simulink library "ammclib_bam"  (Simulink 9.3)
settings: Solver=VariableStepAuto  StartTime=0.0  StopTime=10.0  RelTol=1e-3
undefined symbols (not defined in the file or in its folder): f16A1, f16A2, f16ADCMaxError, f16B0, f16B1, f16B2, f16C1, f16CC1, f16CC1sc, f16CC1sc_D, f16CC1sc_Q, f16CC2, f16CC2sc, f16CC2sc_D, f16CC2sc_Q, f16DerivGain, f16EGain, f16FiltCoef, f16HystOff, f16HystOn, f16IGain, f16IntegGain, f16IntegGainFW, f16IntegGainQ, f16Kd, f16Kq, f16Limit, f16LowerLimit, f16LowerLimit_D, f16LowerLimit_Q, f16LowerLimitFW, f16LowerLimitQ, f16ModIndex, f16OutValOff, f16OutValOn, f16PropGain, f16PropGainFW, f16PropGainQ, f16RampDown, f16RampUp, f16UGain, f16UpperLimit, f16UpperLimit_D, f16UpperLimit_Q, f16UpperLimitFW, f16UpperLimitQ, f16WIGain, f32A1, f32A2, f32ADCMaxError, f32B0, f32B1, f32B2, f32C1, f32CC1, f32CC1sc, f32CC1sc_D, f32CC1sc_Q, f32CC2, f32CC2sc ... (+114)
(part 20 of 21)

== system ammclib_bam/MLIB/F16/MLIB_ShLSat_F16 ==
  f16In1 : Inport  OutDataTypeStr=int16
  u16In2 : Inport  Port=2  OutDataTypeStr=uint16
  MLIB_ShLSat_SF : S-Function  FunctionName=MLIB_ShLSat_SF_F16  SFunctionDeploymentMode=off  EnableBusSupport=off
  copyright : Subsystem
      mask Display: text(10,90,'FILE:');text(10,75,'DESRIPTION:');text(10,60,'COPYRIGHT:');text(10,45,'VERSION:');text(10,30,'DATE:')
  copyright2 : Subsystem
      mask Display: text(10,90,'MLIB_ShLSat_BAM_F16.mdl');text(10,75,'Saturated shift left.');text(10,60,'NXP 2020');text(10,45,'1.0');text(10,30,'18-Mar-2020');
  f16Out : Outport
  wires:
  MLIB_ShLSat_SF/1 -> f16Out/1
  u16In2/1 -> MLIB_ShLSat_SF/2
  f16In1/1 -> MLIB_ShLSat_SF/1

== system ammclib_bam/MLIB/F16/MLIB_ShL_F16 ==
  f16In1 : Inport  OutDataTypeStr=int16
  u16In2 : Inport  Port=2  OutDataTypeStr=uint16
  MLIB_ShL_SF : S-Function  FunctionName=MLIB_ShL_SF_F16  SFunctionDeploymentMode=off  EnableBusSupport=off
  copyright : Subsystem
      mask Display: text(10,90,'FILE:');text(10,75,'DESRIPTION:');text(10,60,'COPYRIGHT:');text(10,45,'VERSION:');text(10,30,'DATE:')
  copyright2 : Subsystem
      mask Display: text(10,90,'MLIB_ShL_BAM_F16.mdl');text(10,75,'Unsaturated shift left.');text(10,60,'NXP 2020');text(10,45,'1.0');text(10,30,'18-Mar-2020');
  f16Out : Outport
  wires:
  MLIB_ShL_SF/1 -> f16Out/1
  u16In2/1 -> MLIB_ShL_SF/2
  f16In1/1 -> MLIB_ShL_SF/1

== system ammclib_bam/MLIB/F16/MLIB_ShR_F16 ==
  f16In1 : Inport  OutDataTypeStr=int16
  u16In2 : Inport  Port=2  OutDataTypeStr=uint16
  MLIB_ShR_SF : S-Function  FunctionName=MLIB_ShR_SF_F16  SFunctionDeploymentMode=off  EnableBusSupport=off
  copyright : Subsystem
      mask Display: text(10,90,'FILE:');text(10,75,'DESRIPTION:');text(10,60,'COPYRIGHT:');text(10,45,'VERSION:');text(10,30,'DATE:')
  copyright2 : Subsystem
      mask Display: text(10,90,'MLIB_ShR_BAM_F16.mdl');text(10,75,'Unsaturated shift right.');text(10,60,'NXP 2020');text(10,45,'1.0');text(10,30,'18-Mar-2020');
  f16Out : Outport
  wires:
  MLIB_ShR_SF/1 -> f16Out/1
  u16In2/1 -> MLIB_ShR_SF/2
  f16In1/1 -> MLIB_ShR_SF/1

== system ammclib_bam/MLIB/F16/MLIB_SubSat_F16 ==
  f16In1 : Inport  OutDataTypeStr=int16
  f16In2 : Inport  Port=2  OutDataTypeStr=int16
  MLIB_SubSat_SF : S-Function  FunctionName=MLIB_SubSat_SF_F16  SFunctionDeploymentMode=off  EnableBusSupport=off
  copyright : Subsystem
      mask Display: text(10,90,'FILE:');text(10,75,'DESRIPTION:');text(10,60,'COPYRIGHT:');text(10,45,'VERSION:');text(10,30,'DATE:')
  copyright2 : Subsystem
      mask Display: text(10,90,'MLIB_SubSat_BAM_F16.mdl');text(10,75,'Saturated subtraction.');text(10,60,'NXP 2020');text(10,45,'1.0');text(10,30,'18-Mar-2020');
  f16Out : Outport
  wires:
  MLIB_SubSat_SF/1 -> f16Out/1
  f16In2/1 -> MLIB_SubSat_SF/2
  f16In1/1 -> MLIB_SubSat_SF/1

== system ammclib_bam/MLIB/F16/MLIB_Sub_F16 ==
  f16In1 : Inport  OutDataTypeStr=int16
  f16In2 : Inport  Port=2  OutDataTypeStr=int16
  MLIB_Sub_SF : S-Function  FunctionName=MLIB_Sub_SF_F16  SFunctionDeploymentMode=off  EnableBusSupport=off
  copyright : Subsystem
      mask Display: text(10,90,'FILE:');text(10,75,'DESRIPTION:');text(10,60,'COPYRIGHT:');text(10,45,'VERSION:');text(10,30,'DATE:')
  copyright2 : Subsystem
      mask Display: text(10,90,'MLIB_Sub_BAM_F16.mdl');text(10,75,'Unsaturated subtraction.');text(10,60,'NXP 2020');text(10,45,'1.0');text(10,30,'18-Mar-2020');
  f16Out : Outport
  wires:
  MLIB_Sub_SF/1 -> f16Out/1
  f16In2/1 -> MLIB_Sub_SF/2
  f16In1/1 -> MLIB_Sub_SF/1

== system ammclib_bam/MLIB/F16/MLIB_VMac_F16 ==
  f16In1 : Inport  OutDataTypeStr=int16
  f16In2 : Inport  Port=2  OutDataTypeStr=int16
  f16In3 : Inport  Port=3  OutDataTypeStr=int16
  f16In4 : Inport  Port=4  OutDataTypeStr=int16
  MLIB_VMac_SF : S-Function  FunctionName=MLIB_VMac_SF_F16  SFunctionDeploymentMode=off  EnableBusSupport=off
  copyright : Subsystem
      mask Display: text(10,90,'FILE:');text(10,75,'DESRIPTION:');text(10,60,'COPYRIGHT:');text(10,45,'VERSION:');text(10,30,'DATE:')
  copyright2 : Subsystem
      mask Display: text(10,90,'MLIB_VMac_BAM_F16.mdl');text(10,75,'Dot product of 2-element vectors with saturated multiplication and modulo accumulation.');text(10,60,'NXP 2020');text(10,45,'1.0');text(10,30,'18-Mar-2020');
  f16Out : Outport
  wires:
  MLIB_VMac_SF/1 -> f16Out/1
  f16In4/1 -> MLIB_VMac_SF/4
  f16In3/1 -> MLIB_VMac_SF/3
  f16In2/1 -> MLIB_VMac_SF/2
  f16In1/1 -> MLIB_VMac_SF/1

== system ammclib_bam/MLIB/F32/MLIB_AbsSat_F32 ==
  f32In : Inport  OutDataTypeStr=int32
  MLIB_AbsSat_SF : S-Function  FunctionName=MLIB_AbsSat_SF_F32  SFunctionDeploymentMode=off  EnableBusSupport=off
  copyright : Subsystem
      mask Display: text(10,90,'FILE:');text(10,75,'DESRIPTION:');text(10,60,'COPYRIGHT:');text(10,45,'VERSION:');text(10,30,'DATE:')
  copyright2 : Subsystem
      mask Display: text(10,90,'MLIB_AbsSat_BAM_F32.mdl');text(10,75,'Saturated absolute value.');text(10,60,'NXP 2020');text(10,45,'1.0');text(10,30,'18-Mar-2020');
  f32Out : Outport
  wires:
  MLIB_AbsSat_SF/1 -> f32Out/1
  f32In/1 -> MLIB_AbsSat_SF/1

== system ammclib_bam/MLIB/F32/MLIB_Abs_F32 ==
  f32In : Inport  OutDataTypeStr=int32
  MLIB_Abs_SF : S-Function  FunctionName=MLIB_Abs_SF_F32  SFunctionDeploymentMode=off  EnableBusSupport=off
  copyright : Subsystem
      mask Display: text(10,90,'FILE:');text(10,75,'DESRIPTION:');text(10,60,'COPYRIGHT:');text(10,45,'VERSION:');text(10,30,'DATE:')
  copyright2 : Subsystem
      mask Display: text(10,90,'MLIB_Abs_BAM_F32.mdl');text(10,75,'Unsaturated absolute value.');text(10,60,'NXP 2020');text(10,45,'1.0');text(10,30,'18-Mar-2020');
  f32Out : Outport
  wires:
  MLIB_Abs_SF/1 -> f32Out/1
  f32In/1 -> MLIB_Abs_SF/1

== system ammclib_bam/MLIB/F32/MLIB_AddSat_F32 ==
  f32In1 : Inport  OutDataTypeStr=int32
  f32In2 : Inport  Port=2  OutDataTypeStr=int32
  MLIB_AddSat_SF : S-Function  FunctionName=MLIB_AddSat_SF_F32  SFunctionDeploymentMode=off  EnableBusSupport=off
  copyright : Subsystem
      mask Display: text(10,90,'FILE:');text(10,75,'DESRIPTION:');text(10,60,'COPYRIGHT:');text(10,45,'VERSION:');text(10,30,'DATE:')
  copyright2 : Subsystem
      mask Display: text(10,90,'MLIB_AddSat_BAM_F32.mdl');text(10,75,'Saturated addition.');text(10,60,'NXP 2020');text(10,45,'1.0');text(10,30,'18-Mar-2020');
  f32Out : Outport
  wires:
  MLIB_AddSat_SF/1 -> f32Out/1
  f32In2/1 -> MLIB_AddSat_SF/2
  f32In1/1 -> MLIB_AddSat_SF/1

== system ammclib_bam/MLIB/F32/MLIB_Add_F32 ==
  f32In1 : Inport  OutDataTypeStr=int32
  f32In2 : Inport  Port=2  OutDataTypeStr=int32
  MLIB_Add_SF : S-Function  FunctionName=MLIB_Add_SF_F32  SFunctionDeploymentMode=off  EnableBusSupport=off
  copyright : Subsystem
      mask Display: text(10,90,'FILE:');text(10,75,'DESRIPTION:');text(10,60,'COPYRIGHT:');text(10,45,'VERSION:');text(10,30,'DATE:')
  copyright2 : Subsystem
      mask Display: text(10,90,'MLIB_Add_BAM_F32.mdl');text(10,75,'Unsaturated addition.');text(10,60,'NXP 2020');text(10,45,'1.0');text(10,30,'18-Mar-2020');
  f32Out : Outport
  wires:
  MLIB_Add_SF/1 -> f32Out/1
  f32In2/1 -> MLIB_Add_SF/2
  f32In1/1 -> MLIB_Add_SF/1

== system ammclib_bam/MLIB/F32/MLIB_ConvertPU_F32F16 ==
  f16In : Inport  OutDataTypeStr=int16
  MLIB_ConvertPU_SF : S-Function  FunctionName=MLIB_ConvertPU_SF_F32F16  SFunctionDeploymentMode=off  EnableBusSupport=off
  copyright : Subsystem
      mask Display: text(10,90,'FILE:');text(10,75,'DESRIPTION:');text(10,60,'COPYRIGHT:');text(10,45,'VERSION:');text(10,30,'DATE:')
  copyright2 : Subsystem
      mask Display: text(10,90,'MLIB_ConvertPU_BAM_F32F16.mdl');text(10,75,'Converts the input value to a different representation.');text(10,60,'NXP 2020');text(10,45,'1.0');text(10,30,'18-Mar-2020');
  f32Out : Outport
  wires:
  MLIB_ConvertPU_SF/1 -> f32Out/1
  f16In/1 -> MLIB_ConvertPU_SF/1

== system ammclib_bam/MLIB/F32/MLIB_ConvertPU_F32FLT ==
  fltIn : Inport  OutDataTypeStr=single
  MLIB_ConvertPU_SF : S-Function  FunctionName=MLIB_ConvertPU_SF_F32FLT  SFunctionDeploymentMode=off  EnableBusSupport=off
  copyright : Subsystem
      mask Display: text(10,90,'FILE:');text(10,75,'DESRIPTION:');text(10,60,'COPYRIGHT:');text(10,45,'VERSION:');text(10,30,'DATE:')
  copyright2 : Subsystem
      mask Display: text(10,90,'MLIB_ConvertPU_BAM_F32FLT.mdl');text(10,75,'Converts the input value to a different representation.');text(10,60,'NXP 2020');text(10,45,'1.0');text(10,30,'18-Mar-2020');
  f32Out : Outport
  wires:
  MLIB_ConvertPU_SF/1 -> f32Out/1
  fltIn/1 -> MLIB_ConvertPU_SF/1

== system ammclib_bam/MLIB/F32/MLIB_Convert_F32F16 ==
  f16In1 : Inport  OutDataTypeStr=int16
  f16In2 : Inport  Port=2  OutDataTypeStr=int16
  MLIB_Convert_SF : S-Function  FunctionName=MLIB_Convert_SF_F32F16  SFunctionDeploymentMode=off  EnableBusSupport=off
  copyright : Subsystem
      mask Display: text(10,90,'FILE:');text(10,75,'DESRIPTION:');text(10,60,'COPYRIGHT:');text(10,45,'VERSION:');text(10,30,'DATE:')
  copyright2 : Subsystem
      mask Display: text(10,90,'MLIB_Convert_BAM_F32F16.mdl');text(10,75,'Converts the input value with scale to a different representation.');text(10,60,'NXP 2020');text(10,45,'1.0');text(10,30,'18-Mar-2020');
  f32Out : Outport
  wires:
  MLIB_Convert_SF/1 -> f32Out/1
  f16In2/1 -> MLIB_Convert_SF/2
  f16In1/1 -> MLIB_Convert_SF/1

== system ammclib_bam/MLIB/F32/MLIB_Convert_F32FLT ==
  fltIn1 : Inport  OutDataTypeStr=single
  fltIn2 : Inport  Port=2  OutDataTypeStr=single
  MLIB_Convert_SF : S-Function  FunctionName=MLIB_Convert_SF_F32FLT  SFunctionDeploymentMode=off  EnableBusSupport=off
  copyright : Subsystem
      mask Display: text(10,90,'FILE:');text(10,75,'DESRIPTION:');text(10,60,'COPYRIGHT:');text(10,45,'VERSION:');text(10,30,'DATE:')
  copyright2 : Subsystem
      mask Display: text(10,90,'MLIB_Convert_BAM_F32FLT.mdl');text(10,75,'Converts the input value with scale to a different representation.');text(10,60,'NXP 2020');text(10,45,'1.0');text(10,30,'18-Mar-2020');
  f32Out : Outport
  wires:
  MLIB_Convert_SF/1 -> f32Out/1
  fltIn2/1 -> MLIB_Convert_SF/2
  fltIn1/1 -> MLIB_Convert_SF/1

== system ammclib_bam/MLIB/F32/MLIB_DivSat_F32 ==
  f32In1 : Inport  OutDataTypeStr=int32
  f32In2 : Inport  Port=2  OutDataTypeStr=int32
  MLIB_DivSat_SF : S-Function  FunctionName=MLIB_DivSat_SF_F32  SFunctionDeploymentMode=off  EnableBusSupport=off
  copyright : Subsystem
      mask Display: text(10,90,'FILE:');text(10,75,'DESRIPTION:');text(10,60,'COPYRIGHT:');text(10,45,'VERSION:');text(10,30,'DATE:')
  copyright2 : Subsystem
      mask Display: text(10,90,'MLIB_DivSat_BAM_F32.mdl');text(10,75,'Saturated division.');text(10,60,'NXP 2020');text(10,45,'1.0');text(10,30,'18-Mar-2020');
  f32Out : Outport
  wires:
  MLIB_DivSat_SF/1 -> f32Out/1
  f32In2/1 -> MLIB_DivSat_SF/2
  f32In1/1 -> MLIB_DivSat_SF/1

== system ammclib_bam/MLIB/F32/MLIB_Div_F32 ==
  f32In1 : Inport  OutDataTypeStr=int32
  f32In2 : Inport  Port=2  OutDataTypeStr=int32
  MLIB_Div_SF : S-Function  FunctionName=MLIB_Div_SF_F32  SFunctionDeploymentMode=off  EnableBusSupport=off
  copyright : Subsystem
      mask Display: text(10,90,'FILE:');text(10,75,'DESRIPTION:');text(10,60,'COPYRIGHT:');text(10,45,'VERSION:');text(10,30,'DATE:')
  copyright2 : Subsystem
      mask Display: text(10,90,'MLIB_Div_BAM_F32.mdl');text(10,75,'Division of two input values.');text(10,60,'NXP 2020');text(10,45,'1.0');text(10,30,'18-Mar-2020');
  f32Out : Outport
  wires:
  MLIB_Div_SF/1 -> f32Out/1
  f32In2/1 -> MLIB_Div_SF/2
  f32In1/1 -> MLIB_Div_SF/1

== system ammclib_bam/MLIB/F32/MLIB_MacSat_F32 ==
  f32In1 : Inport  OutDataTypeStr=int32
  f32In2 : Inport  Port=2  OutDataTypeStr=int32
  f32In3 : Inport  Port=3  OutDataTypeStr=int32
  MLIB_MacSat_SF : S-Function  FunctionName=MLIB_MacSat_SF_F32  SFunctionDeploymentMode=off  EnableBusSupport=off
  copyright : Subsystem
      mask Display: text(10,90,'FILE:');text(10,75,'DESRIPTION:');text(10,60,'COPYRIGHT:');text(10,45,'VERSION:');text(10,30,'DATE:')
  copyright2 : Subsystem
      mask Display: text(10,90,'MLIB_MacSat_BAM_F32.mdl');text(10,75,'Saturated multiply-accumulate.');text(10,60,'NXP 2020');text(10,45,'1.0');text(10,30,'18-Mar-2020');
  f32Out : Outport
  wires:
  MLIB_MacSat_SF/1 -> f32Out/1
  f32In3/1 -> MLIB_MacSat_SF/3
  f32In2/1 -> MLIB_MacSat_SF/2
  f32In1/1 -> MLIB_MacSat_SF/1

== system ammclib_bam/MLIB/F32/MLIB_Mac_F32 ==
  f32In1 : Inport  OutDataTypeStr=int32
  f32In2 : Inport  Port=2  OutDataTypeStr=int32
  f32In3 : Inport  Port=3  OutDataTypeStr=int32
  MLIB_Mac_SF : S-Function  FunctionName=MLIB_Mac_SF_F32  SFunctionDeploymentMode=off  EnableBusSupport=off
  copyright : Subsystem
      mask Display: text(10,90,'FILE:');text(10,75,'DESRIPTION:');text(10,60,'COPYRIGHT:');text(10,45,'VERSION:');text(10,30,'DATE:')
  copyright2 : Subsystem
      mask Display: text(10,90,'MLIB_Mac_BAM_F32.mdl');text(10,75,'Multiply-accumulte.');text(10,60,'NXP 2020');text(10,45,'1.0');text(10,30,'18-Mar-2020');
  f32Out : Outport
  wires:
  MLIB_Mac_SF/1 -> f32Out/1
  f32In3/1 -> MLIB_Mac_SF/3
  f32In2/1 -> MLIB_Mac_SF/2
  f32In1/1 -> MLIB_Mac_SF/1

== system ammclib_bam/MLIB/F32/MLIB_Mnac_F32 ==
  f32In1 : Inport  OutDataTypeStr=int32
  f32In2 : Inport  Port=2  OutDataTypeStr=int32
  f32In3 : Inport  Port=3  OutDataTypeStr=int32
  MLIB_Mnac_SF : S-Function  FunctionName=MLIB_Mnac_SF_F32  SFunctionDeploymentMode=off  EnableBusSupport=off
  copyright : Subsystem
      mask Display: text(10,90,'FILE:');text(10,75,'DESRIPTION:');text(10,60,'COPYRIGHT:');text(10,45,'VERSION:');text(10,30,'DATE:')
  copyright2 : Subsystem
      mask Display: text(10,90,'MLIB_Mnac_BAM_F32.mdl');text(10,75,'Unsaturated multiply-negative-accumulate.');text(10,60,'NXP 2020');text(10,45,'1.0');text(10,30,'18-Mar-2020');
  f32Out : Outport
  wires:
  MLIB_Mnac_SF/1 -> f32Out/1
  f32In3/1 -> MLIB_Mnac_SF/3
  f32In2/1 -> MLIB_Mnac_SF/2
  f32In1/1 -> MLIB_Mnac_SF/1

== system ammclib_bam/MLIB/F32/MLIB_Msu_F32 ==
  f32In1 : Inport  OutDataTypeStr=int32
  f32In2 : Inport  Port=2  OutDataTypeStr=int32
  f32In3 : Inport  Port=3  OutDataTypeStr=int32
  MLIB_Msu_SF : S-Function  FunctionName=MLIB_Msu_SF_F32  SFunctionDeploymentMode=off  EnableBusSupport=off
  copyright : Subsystem
      mask Display: text(10,90,'FILE:');text(10,75,'DESRIPTION:');text(10,60,'COPYRIGHT:');text(10,45,'VERSION:');text(10,30,'DATE:')
  copyright2 : Subsystem
      mask Display: text(10,90,'MLIB_Msu_BAM_F32.mdl');text(10,75,'Unsaturated multiply-subtract-from.');text(10,60,'NXP 2020');text(10,45,'1.0');text(10,30,'18-Mar-2020');
  f32Out : Outport
  wires:
  MLIB_Msu_SF/1 -> f32Out/1
  f32In3/1 -> MLIB_Msu_SF/3
  f32In2/1 -> MLIB_Msu_SF/2
  f32In1/1 -> MLIB_Msu_SF/1

== system ammclib_bam/MLIB/F32/MLIB_MulSat_F32 ==
  f32In1 : Inport  OutDataTypeStr=int32
  f32In2 : Inport  Port=2  OutDataTypeStr=int32
  MLIB_MulSat_SF : S-Function  FunctionName=MLIB_MulSat_SF_F32  SFunctionDeploymentMode=off  EnableBusSupport=off
  copyright : Subsystem
      mask Display: text(10,90,'FILE:');text(10,75,'DESRIPTION:');text(10,60,'COPYRIGHT:');text(10,45,'VERSION:');text(10,30,'DATE:')
  copyright2 : Subsystem
      mask Display: text(10,90,'MLIB_MulSat_BAM_F32.mdl');text(10,75,'Saturated multiplication.');text(10,60,'NXP 2020');text(10,45,'1.0');text(10,30,'18-Mar-2020');
  f32Out : Outport
  wires:
  MLIB_MulSat_SF/1 -> f32Out/1
  f32In2/1 -> MLIB_MulSat_SF/2
  f32In1/1 -> MLIB_MulSat_SF/1

== system ammclib_bam/MLIB/F32/MLIB_Mul_F32 ==
  f32In1 : Inport  OutDataTypeStr=int32
  f32In2 : Inport  Port=2  OutDataTypeStr=int32
  MLIB_Mul_SF : S-Function  FunctionName=MLIB_Mul_SF_F32  SFunctionDeploymentMode=off  EnableBusSupport=off
  copyright : Subsystem
      mask Display: text(10,90,'FILE:');text(10,75,'DESRIPTION:');text(10,60,'COPYRIGHT:');text(10,45,'VERSION:');text(10,30,'DATE:')
  copyright2 : Subsystem
      mask Display: text(10,90,'MLIB_Mul_BAM_F32.mdl');text(10,75,'Unsaturated multiplication.');text(10,60,'NXP 2020');text(10,45,'1.0');text(10,30,'18-Mar-2020');
  f32Out : Outport
  wires:
  MLIB_Mul_SF/1 -> f32Out/1
  f32In2/1 -> MLIB_Mul_SF/2
  f32In1/1 -> MLIB_Mul_SF/1

== system ammclib_bam/MLIB/F32/MLIB_NegSat_F32 ==
  f32In : Inport  OutDataTypeStr=int32
  MLIB_NegSat_SF : S-Function  FunctionName=MLIB_NegSat_SF_F32  SFunctionDeploymentMode=off  EnableBusSupport=off
  copyright : Subsystem
      mask Display: text(10,90,'FILE:');text(10,75,'DESRIPTION:');text(10,60,'COPYRIGHT:');text(10,45,'VERSION:');text(10,30,'DATE:')
  copyright2 : Subsystem
      mask Display: text(10,90,'MLIB_NegSat_BAM_F32.mdl');text(10,75,'Saturated negation.');text(10,60,'NXP 2020');text(10,45,'1.0');text(10,30,'18-Mar-2020');
  f32Out : Outport
  wires:
  MLIB_NegSat_SF/1 -> f32Out/1
  f32In/1 -> MLIB_NegSat_SF/1

== system ammclib_bam/MLIB/F32/MLIB_Neg_F32 ==
  f32In : Inport  OutDataTypeStr=int32
  MLIB_Neg_SF : S-Function  FunctionName=MLIB_Neg_SF_F32  SFunctionDeploymentMode=off  EnableBusSupport=off
  copyright : Subsystem
      mask Display: text(10,90,'FILE:');text(10,75,'DESRIPTION:');text(10,60,'COPYRIGHT:');text(10,45,'VERSION:');text(10,30,'DATE:')
  copyright2 : Subsystem
      mask Display: text(10,90,'MLIB_Neg_BAM_F32.mdl');text(10,75,'Unsaturated negation.');text(10,60,'NXP 2020');text(10,45,'1.0');text(10,30,'18-Mar-2020');
  f32Out : Outport
  wires:
  MLIB_Neg_SF/1 -> f32Out/1
  f32In/1 -> MLIB_Neg_SF/1

== system ammclib_bam/MLIB/F32/MLIB_Norm_F32 ==
  f32In : Inport  OutDataTypeStr=int32
  MLIB_Norm_SF : S-Function  FunctionName=MLIB_Norm_SF_F32  SFunctionDeploymentMode=off  EnableBusSupport=off
  copyright : Subsystem
      mask Display: text(10,90,'FILE:');text(10,75,'DESRIPTION:');text(10,60,'COPYRIGHT:');text(10,45,'VERSION:');text(10,30,'DATE:')
  copyright2 : Subsystem
      mask Display: text(10,90,'MLIB_Norm_BAM_F32.mdl');text(10,75,'Normalization of the input value.');text(10,60,'NXP 2020');text(10,45,'1.0');text(10,30,'18-Mar-2020');
  u16Out : Outport
  wires:
  MLIB_Norm_SF/1 -> u16Out/1
  f32In/1 -> MLIB_Norm_SF/1

== system ammclib_bam/MLIB/F32/MLIB_Round_F32 ==
  f32In1 : Inport  OutDataTypeStr=int32
  u16In2 : Inport  Port=2  OutDataTypeStr=uint16
  MLIB_Round_SF : S-Function  FunctionName=MLIB_Round_SF_F32  SFunctionDeploymentMode=off  EnableBusSupport=off
  copyright : Subsystem
      mask Display: text(10,90,'FILE:');text(10,75,'DESRIPTION:');text(10,60,'COPYRIGHT:');text(10,45,'VERSION:');text(10,30,'DATE:')
  copyright2 : Subsystem
      mask Display: text(10,90,'MLIB_Round_BAM_F32.mdl');text(10,75,'Round the first input value.');text(10,60,'NXP 2020');text(10,45,'1.0');text(10,30,'18-Mar-2020');
  f32Out : Outport
  wires:
  MLIB_Round_SF/1 -> f32Out/1
  u16In2/1 -> MLIB_Round_SF/2
  f32In1/1 -> MLIB_Round_SF/1

== system ammclib_bam/MLIB/F32/MLIB_ShBiSat_F32 ==
  f32In1 : Inport  OutDataTypeStr=int32
  s16In2 : Inport  Port=2  OutDataTypeStr=int16
  MLIB_ShBiSat_SF : S-Function  FunctionName=MLIB_ShBiSat_SF_F32  SFunctionDeploymentMode=off  EnableBusSupport=off
  copyright : Subsystem
      mask Display: text(10,90,'FILE:');text(10,75,'DESRIPTION:');text(10,60,'COPYRIGHT:');text(10,45,'VERSION:');text(10,30,'DATE:')
  copyright2 : Subsystem
      mask Display: text(10,90,'MLIB_ShBiSat_BAM_F32.mdl');text(10,75,'Saturated bidirectional shift.');text(10,60,'NXP 2020');text(10,45,'1.0');text(10,30,'18-Mar-2020');
  f32Out : Outport
  wires:
  MLIB_ShBiSat_SF/1 -> f32Out/1
  s16In2/1 -> MLIB_ShBiSat_SF/2
  f32In1/1 -> MLIB_ShBiSat_SF/1

== system ammclib_bam/MLIB/F32/MLIB_ShBi_F32 ==
  f32In1 : Inport  OutDataTypeStr=int32
  s16In2 : Inport  Port=2  OutDataTypeStr=int16
  MLIB_ShBi_SF : S-Function  FunctionName=MLIB_ShBi_SF_F32  SFunctionDeploymentMode=off  EnableBusSupport=off
  copyright : Subsystem
      mask Display: text(10,90,'FILE:');text(10,75,'DESRIPTION:');text(10,60,'COPYRIGHT:');text(10,45,'VERSION:');text(10,30,'DATE:')
  copyright2 : Subsystem
      mask Display: text(10,90,'MLIB_ShBi_BAM_F32.mdl');text(10,75,'Unsaturated bidirectional shift.');text(10,60,'NXP 2020');text(10,45,'1.0');text(10,30,'18-Mar-2020');
  f32Out : Outport
  wires:
  MLIB_ShBi_SF/1 -> f32Out/1
  s16In2/1 -> MLIB_ShBi_SF/2
  f32In1/1 -> MLIB_ShBi_SF/1

== system ammclib_bam/MLIB/F32/MLIB_ShLSat_F32 ==
  f32In1 : Inport  OutDataTypeStr=int32
  u16In2 : Inport  Port=2  OutDataTypeStr=uint16
  MLIB_ShLSat_SF : S-Function  FunctionName=MLIB_ShLSat_SF_F32  SFunctionDeploymentMode=off  EnableBusSupport=off
  copyright : Subsystem
      mask Display: text(10,90,'FILE:');text(10,75,'DESRIPTION:');text(10,60,'COPYRIGHT:');text(10,45,'VERSION:');text(10,30,'DATE:')
  copyright2 : Subsystem
      mask Display: text(10,90,'MLIB_ShLSat_BAM_F32.mdl');text(10,75,'Saturated shift left.');text(10,60,'NXP 2020');text(10,45,'1.0');text(10,30,'18-Mar-2020');
  f32Out : Outport
  wires:
  MLIB_ShLSat_SF/1 -> f32Out/1
  u16In2/1 -> MLIB_ShLSat_SF/2
  f32In1/1 -> MLIB_ShLSat_SF/1

== system ammclib_bam/MLIB/F32/MLIB_ShL_F32 ==
  f32In1 : Inport  OutDataTypeStr=int32
  u16In2 : Inport  Port=2  OutDataTypeStr=uint16
  MLIB_ShL_SF : S-Function  FunctionName=MLIB_ShL_SF_F32  SFunctionDeploymentMode=off  EnableBusSupport=off
  copyright : Subsystem
      mask Display: text(10,90,'FILE:');text(10,75,'DESRIPTION:');text(10,60,'COPYRIGHT:');text(10,45,'VERSION:');text(10,30,'DATE:')
  copyright2 : Subsystem
      mask Display: text(10,90,'MLIB_ShL_BAM_F32.mdl');text(10,75,'Unsaturated shift left.');text(10,60,'NXP 2020');text(10,45,'1.0');text(10,30,'18-Mar-2020');
  f32Out : Outport
  wires:
  MLIB_ShL_SF/1 -> f32Out/1
  u16In2/1 -> MLIB_ShL_SF/2
  f32In1/1 -> MLIB_ShL_SF/1

== system ammclib_bam/MLIB/F32/MLIB_ShR_F32 ==
  f32In1 : Inport  OutDataTypeStr=int32
  u16In2 : Inport  Port=2  OutDataTypeStr=uint16
  MLIB_ShR_SF : S-Function  FunctionName=MLIB_ShR_SF_F32  SFunctionDeploymentMode=off  EnableBusSupport=off
  copyright : Subsystem
      mask Display: text(10,90,'FILE:');text(10,75,'DESRIPTION:');text(10,60,'COPYRIGHT:');text(10,45,'VERSION:');text(10,30,'DATE:')
  copyright2 : Subsystem
      mask Display: text(10,90,'MLIB_ShR_BAM_F32.mdl');text(10,75,'Unsaturated shift right.');text(10,60,'NXP 2020');text(10,45,'1.0');text(10,30,'18-Mar-2020');
  f32Out : Outport
  wires:
  MLIB_ShR_SF/1 -> f32Out/1
  u16In2/1 -> MLIB_ShR_SF/2
  f32In1/1 -> MLIB_ShR_SF/1

== system ammclib_bam/MLIB/F32/MLIB_SubSat_F32 ==
  f32In1 : Inport  OutDataTypeStr=int32
  f32In2 : Inport  Port=2  OutDataTypeStr=int32
  MLIB_SubSat_SF : S-Function  FunctionName=MLIB_SubSat_SF_F32  SFunctionDeploymentMode=off  EnableBusSupport=off
  copyright : Subsystem
      mask Display: text(10,90,'FILE:');text(10,75,'DESRIPTION:');text(10,60,'COPYRIGHT:');text(10,45,'VERSION:');text(10,30,'DATE:')
  copyright2 : Subsystem
      mask Display: text(10,90,'MLIB_SubSat_BAM_F32.mdl');text(10,75,'Saturated subtraction.');text(10,60,'NXP 2020');text(10,45,'1.0');text(10,30,'18-Mar-2020');
  f32Out : Outport
  wires:
  MLIB_SubSat_SF/1 -> f32Out/1
  f32In2/1 -> MLIB_SubSat_SF/2
  f32In1/1 -> MLIB_SubSat_SF/1

== system ammclib_bam/MLIB/F32/MLIB_Sub_F32 ==
  f32In1 : Inport  OutDataTypeStr=int32
  f32In2 : Inport  Port=2  OutDataTypeStr=int32
  MLIB_Sub_SF : S-Function  FunctionName=MLIB_Sub_SF_F32  SFunctionDeploymentMode=off  EnableBusSupport=off
  copyright : Subsystem
      mask Display: text(10,90,'FILE:');text(10,75,'DESRIPTION:');text(10,60,'COPYRIGHT:');text(10,45,'VERSION:');text(10,30,'DATE:')
  copyright2 : Subsystem
      mask Display: text(10,90,'MLIB_Sub_BAM_F32.mdl');text(10,75,'Unsaturated subtraction.');text(10,60,'NXP 2020');text(10,45,'1.0');text(10,30,'18-Mar-2020');
  f32Out : Outport
  wires:
  MLIB_Sub_SF/1 -> f32Out/1
  f32In2/1 -> MLIB_Sub_SF/2
  f32In1/1 -> MLIB_Sub_SF/1

== system ammclib_bam/MLIB/F32/MLIB_VMac_F32 ==
  f32In1 : Inport  OutDataTypeStr=int32
  f32In2 : Inport  Port=2  OutDataTypeStr=int32
  f32In3 : Inport  Port=3  OutDataTypeStr=int32
  f32In4 : Inport  Port=4  OutDataTypeStr=int32
  MLIB_VMac_SF : S-Function  FunctionName=MLIB_VMac_SF_F32  SFunctionDeploymentMode=off  EnableBusSupport=off
  copyright : Subsystem
      mask Display: text(10,90,'FILE:');text(10,75,'DESRIPTION:');text(10,60,'COPYRIGHT:');text(10,45,'VERSION:');text(10,30,'DATE:')
  copyright2 : Subsystem
      mask Display: text(10,90,'MLIB_VMac_BAM_F32.mdl');text(10,75,'Dot product of 2-element vectors with saturated multiplication and modulo accumulation.');text(10,60,'NXP 2020');text(10,45,'1.0');text(10,30,'18-Mar-2020');
  f32Out : Outport
  wires:
  MLIB_VMac_SF/1 -> f32Out/1
  f32In4/1 -> MLIB_VMac_SF/4
  f32In3/1 -> MLIB_VMac_SF/3
  f32In2/1 -> MLIB_VMac_SF/2
  f32In1/1 -> MLIB_VMac_SF/1

== system ammclib_bam/MLIB/F32F16F16/MLIB_MacSat_F32F16F16 ==
  f32In1 : Inport  OutDataTypeStr=int32
  f16In2 : Inport  Port=2  OutDataTypeStr=int16
  f16In3 : Inport  Port=3  OutDataTypeStr=int16
  MLIB_MacSat_SF : S-Function  FunctionName=MLIB_MacSat_SF_F32F16F16  SFunctionDeploymentMode=off  EnableBusSupport=off
  copyright : Subsystem
      mask Display: text(10,90,'FILE:');text(10,75,'DESRIPTION:');text(10,60,'COPYRIGHT:');text(10,45,'VERSION:');text(10,30,'DATE:')
  copyright2 : Subsystem
      mask Display: text(10,90,'MLIB_MacSat_BAM_F32F16F16.mdl');text(10,75,'Saturated multiply-accumulate.');text(10,60,'NXP 2020');text(10,45,'1.0');text(10,30,'18-Mar-2020');
  f32Out : Outport
  wires:
  MLIB_MacSat_SF/1 -> f32Out/1
  f16In3/1 -> MLIB_MacSat_SF/3
  f16In2/1 -> MLIB_MacSat_SF/2
  f32In1/1 -> MLIB_MacSat_SF/1

== system ammclib_bam/MLIB/F32F16F16/MLIB_Mac_F32F16F16 ==
  f32In1 : Inport  OutDataTypeStr=int32
  f16In2 : Inport  Port=2  OutDataTypeStr=int16
  f16In3 : Inport  Port=3  OutDataTypeStr=int16
  MLIB_Mac_SF : S-Function  FunctionName=MLIB_Mac_SF_F32F16F16  SFunctionDeploymentMode=off  EnableBusSupport=off
  copyright : Subsystem
      mask Display: text(10,90,'FILE:');text(10,75,'DESRIPTION:');text(10,60,'COPYRIGHT:');text(10,45,'VERSION:');text(10,30,'DATE:')
  copyright2 : Subsystem
      mask Display: text(10,90,'MLIB_Mac_BAM_F32F16F16.mdl');text(10,75,'Multiply-accumulte.');text(10,60,'NXP 2020');text(10,45,'1.0');text(10,30,'18-Mar-2020');
  f32Out : Outport
  wires:
  MLIB_Mac_SF/1 -> f32Out/1
  f16In3/1 -> MLIB_Mac_SF/3
  f16In2/1 -> MLIB_Mac_SF/2
  f32In1/1 -> MLIB_Mac_SF/1

== system ammclib_bam/MLIB/F32F16F16/MLIB_Mnac_F32F16F16 ==
  f32In1 : Inport  OutDataTypeStr=int32
  f16In2 : Inport  Port=2  OutDataTypeStr=int16
  f16In3 : Inport  Port=3  OutDataTypeStr=int16
  MLIB_Mnac_SF : S-Function  FunctionName=MLIB_Mnac_SF_F32F16F16  SFunctionDeploymentMode=off  EnableBusSupport=off
  copyright : Subsystem
      mask Display: text(10,90,'FILE:');text(10,75,'DESRIPTION:');text(10,60,'COPYRIGHT:');text(10,45,'VERSION:');text(10,30,'DATE:')
  copyright2 : Subsystem
      mask Display: text(10,90,'MLIB_Mnac_BAM_F32F16F16.mdl');text(10,75,'Unsaturated multiply-negative-accumulate.');text(10,60,'NXP 2020');text(10,45,'1.0');text(10,30,'18-Mar-2020');
  f32Out : Outport
  wires:
  MLIB_Mnac_SF/1 -> f32Out/1
  f16In3/1 -> MLIB_Mnac_SF/3
  f16In2/1 -> MLIB_Mnac_SF/2
  f32In1/1 -> MLIB_Mnac_SF/1

== system ammclib_bam/MLIB/F32F16F16/MLIB_Msu_F32F16F16 ==
  f32In1 : Inport  OutDataTypeStr=int32
  f16In2 : Inport  Port=2  OutDataTypeStr=int16
  f16In3 : Inport  Port=3  OutDataTypeStr=int16
  MLIB_Msu_SF : S-Function  FunctionName=MLIB_Msu_SF_F32F16F16  SFunctionDeploymentMode=off  EnableBusSupport=off
  copyright : Subsystem
      mask Display: text(10,90,'FILE:');text(10,75,'DESRIPTION:');text(10,60,'COPYRIGHT:');text(10,45,'VERSION:');text(10,30,'DATE:')
  copyright2 : Subsystem
      mask Display: text(10,90,'MLIB_Msu_BAM_F32F16F16.mdl');text(10,75,'Unsaturated multiply-subtract-from.');text(10,60,'NXP 2020');text(10,45,'1.0');text(10,30,'18-Mar-2020');
  f32Out : Outport
  wires:
  MLIB_Msu_SF/1 -> f32Out/1
  f16In3/1 -> MLIB_Msu_SF/3
  f16In2/1 -> MLIB_Msu_SF/2
  f32In1/1 -> MLIB_Msu_SF/1

== system ammclib_bam/MLIB/F32F16F16/MLIB_MulSat_F32F16F16 ==
  f16In1 : Inport  OutDataTypeStr=int16
  f16In2 : Inport  Port=2  OutDataTypeStr=int16
  MLIB_MulSat_SF : S-Function  FunctionName=MLIB_MulSat_SF_F32F16F16  SFunctionDeploymentMode=off  EnableBusSupport=off
  copyright : Subsystem
      mask Display: text(10,90,'FILE:');text(10,75,'DESRIPTION:');text(10,60,'COPYRIGHT:');text(10,45,'VERSION:');text(10,30,'DATE:')
  copyright2 : Subsystem
      mask Display: text(10,90,'MLIB_MulSat_BAM_F32F16F16.mdl');text(10,75,'Saturated multiplication.');text(10,60,'NXP 2020');text(10,45,'1.0');text(10,30,'18-Mar-2020');
  f32Out : Outport
  wires:
  MLIB_MulSat_SF/1 -> f32Out/1
  f16In2/1 -> MLIB_MulSat_SF/2
  f16In1/1 -> MLIB_MulSat_SF/1

== system ammclib_bam/MLIB/F32F16F16/MLIB_Mul_F32F16F16 ==
  f16In1 : Inport  OutDataTypeStr=int16
  f16In2 : Inport  Port=2  OutDataTypeStr=int16
  MLIB_Mul_SF : S-Function  FunctionName=MLIB_Mul_SF_F32F16F16  SFunctionDeploymentMode=off  EnableBusSupport=off
  copyright : Subsystem
      mask Display: text(10,90,'FILE:');text(10,75,'DESRIPTION:');text(10,60,'COPYRIGHT:');text(10,45,'VERSION:');text(10,30,'DATE:')
  copyright2 : Subsystem
      mask Display: text(10,90,'MLIB_Mul_BAM_F32F16F16.mdl');text(10,75,'Unsaturated multiplication.');text(10,60,'NXP 2020');text(10,45,'1.0');text(10,30,'18-Mar-2020');
  f32Out : Outport
  wires:
  MLIB_Mul_SF/1 -> f32Out/1
  f16In2/1 -> MLIB_Mul_SF/2
  f16In1/1 -> MLIB_Mul_SF/1

== system ammclib_bam/MLIB/F32F16F16/MLIB_VMac_F32F16F16 ==
  f16In1 : Inport  OutDataTypeStr=int16
  f16In2 : Inport  Port=2  OutDataTypeStr=int16
  f16In3 : Inport  Port=3  OutDataTypeStr=int16
  f16In4 : Inport  Port=4  OutDataTypeStr=int16
  MLIB_VMac_SF : S-Function  FunctionName=MLIB_VMac_SF_F32F16F16  SFunctionDeploymentMode=off  EnableBusSupport=off
  copyright : Subsystem
      mask Display: text(10,90,'FILE:');text(10,75,'DESRIPTION:');text(10,60,'COPYRIGHT:');text(10,45,'VERSION:');text(10,30,'DATE:')
  copyright2 : Subsystem
      mask Display: text(10,90,'MLIB_VMac_BAM_F32F16F16.mdl');text(10,75,'Dot product of 2-element vectors with saturated multiplication and modulo accumulation.');text(10,60,'NXP 2020');text(10,45,'1.0');text(10,30,'18-Mar-2020');
  f32Out : Outport
  wires:
  MLIB_VMac_SF/1 -> f32Out/1
  f16In4/1 -> MLIB_VMac_SF/4
  f16In3/1 -> MLIB_VMac_SF/3
  f16In2/1 -> MLIB_VMac_SF/2
  f16In1/1 -> MLIB_VMac_SF/1

== system ammclib_bam/MLIB/FLT/MLIB_Abs_FLT ==
  fltIn : Inport  OutDataTypeStr=single
  MLIB_Abs_SF : S-Function  FunctionName=MLIB_Abs_SF_FLT  SFunctionDeploymentMode=off  EnableBusSupport=off
  copyright : Subsystem
      mask Display: text(10,90,'FILE:');text(10,75,'DESRIPTION:');text(10,60,'COPYRIGHT:');text(10,45,'VERSION:');text(10,30,'DATE:')
  copyright2 : Subsystem
      mask Display: text(10,90,'MLIB_Abs_BAM_FLT.mdl');text(10,75,'Absolute value.');text(10,60,'NXP 2020');text(10,45,'1.0');text(10,30,'18-Mar-2020');
  fltOut : Outport
  wires:
  MLIB_Abs_SF/1 -> fltOut/1
  fltIn/1 -> MLIB_Abs_SF/1

== system ammclib_bam/MLIB/FLT/MLIB_Add_FLT ==
  fltIn1 : Inport  OutDataTypeStr=single
  fltIn2 : Inport  Port=2  OutDataTypeStr=single
  MLIB_Add_SF : S-Function  FunctionName=MLIB_Add_SF_FLT  SFunctionDeploymentMode=off  EnableBusSupport=off
  copyright : Subsystem
      mask Display: text(10,90,'FILE:');text(10,75,'DESRIPTION:');text(10,60,'COPYRIGHT:');text(10,45,'VERSION:');text(10,30,'DATE:')
  copyright2 : Subsystem
      mask Display: text(10,90,'MLIB_Add_BAM_FLT.mdl');text(10,75,'Addition.');text(10,60,'NXP 2020');text(10,45,'1.0');text(10,30,'18-Mar-2020');
  fltOut : Outport
  wires:
  MLIB_Add_SF/1 -> fltOut/1
  fltIn2/1 -> MLIB_Add_SF/2
  fltIn1/1 -> MLIB_Add_SF/1

== system ammclib_bam/MLIB/FLT/MLIB_ConvertPU_FLTF16 ==
  f16In : Inport  OutDataTypeStr=int16
  MLIB_ConvertPU_SF : S-Function  FunctionName=MLIB_ConvertPU_SF_FLTF16  SFunctionDeploymentMode=off  EnableBusSupport=off
  copyright : Subsystem
      mask Display: text(10,90,'FILE:');text(10,75,'DESRIPTION:');text(10,60,'COPYRIGHT:');text(10,45,'VERSION:');text(10,30,'DATE:')
  copyright2 : Subsystem
      mask Display: text(10,90,'MLIB_ConvertPU_BAM_FLTF16.mdl');text(10,75,'Converts the input value to a different representation.');text(10,60,'NXP 2020');text(10,45,'1.0');text(10,30,'18-Mar-2020');
  fltOut : Outport
  wires:
  MLIB_ConvertPU_SF/1 -> fltOut/1
  f16In/1 -> MLIB_ConvertPU_SF/1

== system ammclib_bam/MLIB/FLT/MLIB_ConvertPU_FLTF32 ==
  f32In : Inport  OutDataTypeStr=int32
  MLIB_ConvertPU_SF : S-Function  FunctionName=MLIB_ConvertPU_SF_FLTF32  SFunctionDeploymentMode=off  EnableBusSupport=off
  copyright : Subsystem
      mask Display: text(10,90,'FILE:');text(10,75,'DESRIPTION:');text(10,60,'COPYRIGHT:');text(10,45,'VERSION:');text(10,30,'DATE:')
  copyright2 : Subsystem
      mask Display: text(10,90,'MLIB_ConvertPU_BAM_FLTF32.mdl');text(10,75,'Converts the input value to a different representation.');text(10,60,'NXP 2020');text(10,45,'1.0');text(10,30,'18-Mar-2020');
  fltOut : Outport
  wires:
  MLIB_ConvertPU_SF/1 -> fltOut/1
  f32In/1 -> MLIB_ConvertPU_SF/1

== system ammclib_bam/MLIB/FLT/MLIB_Convert_FLTF16 ==
  f16In1 : Inport  OutDataTypeStr=int16
  f16In2 : Inport  Port=2  OutDataTypeStr=int16
  MLIB_Convert_SF : S-Function  FunctionName=MLIB_Convert_SF_FLTF16  SFunctionDeploymentMode=off  EnableBusSupport=off
  copyright : Subsystem
      mask Display: text(10,90,'FILE:');text(10,75,'DESRIPTION:');text(10,60,'COPYRIGHT:');text(10,45,'VERSION:');text(10,30,'DATE:')
  copyright2 : Subsystem
      mask Display: text(10,90,'MLIB_Convert_BAM_FLTF16.mdl');text(10,75,'Converts the input value with scale to a different representation.');text(10,60,'NXP 2020');text(10,45,'1.0');text(10,30,'18-Mar-2020');
  fltOut : Outport
  wires:
  MLIB_Convert_SF/1 -> fltOut/1
  f16In2/1 -> MLIB_Convert_SF/2
  f16In1/1 -> MLIB_Convert_SF/1

== system ammclib_bam/MLIB/FLT/MLIB_Convert_FLTF32 ==
  f32In1 : Inport  OutDataTypeStr=int32
  f32In2 : Inport  Port=2  OutDataTypeStr=int32
  MLIB_Convert_SF : S-Function  FunctionName=MLIB_Convert_SF_FLTF32  SFunctionDeploymentMode=off  EnableBusSupport=off
  copyright : Subsystem
      mask Display: text(10,90,'FILE:');text(10,75,'DESRIPTION:');text(10,60,'COPYRIGHT:');text(10,45,'VERSION:');text(10,30,'DATE:')
  copyright2 : Subsystem
      mask Display: text(10,90,'MLIB_Convert_BAM_FLTF32.mdl');text(10,75,'Converts the input value with scale to a different representation.');text(10,60,'NXP 2020');text(10,45,'1.0');text(10,30,'18-Mar-2020');
  fltOut : Outport
  wires:
  MLIB_Convert_SF/1 -> fltOut/1
  f32In2/1 -> MLIB_Convert_SF/2
  f32In1/1 -> MLIB_Convert_SF/1

== system ammclib_bam/MLIB/FLT/MLIB_Div_FLT ==
  fltIn1 : Inport  OutDataTypeStr=single
  fltIn2 : Inport  Port=2  OutDataTypeStr=single
  MLIB_Div_SF : S-Function  FunctionName=MLIB_Div_SF_FLT  SFunctionDeploymentMode=off  EnableBusSupport=off
  copyright : Subsystem
      mask Display: text(10,90,'FILE:');text(10,75,'DESRIPTION:');text(10,60,'COPYRIGHT:');text(10,45,'VERSION:');text(10,30,'DATE:')
  copyright2 : Subsystem
      mask Display: text(10,90,'MLIB_Div_BAM_FLT.mdl');text(10,75,'Division of two input values.');text(10,60,'NXP 2020');text(10,45,'1.0');text(10,30,'18-Mar-2020');
  fltOut : Outport
  wires:
  MLIB_Div_SF/1 -> fltOut/1
  fltIn2/1 -> MLIB_Div_SF/2
  fltIn1/1 -> MLIB_Div_SF/1

== system ammclib_bam/MLIB/FLT/MLIB_Mac_FLT ==
  fltIn1 : Inport  OutDataTypeStr=single
  fltIn2 : Inport  Port=2  OutDataTypeStr=single
  fltIn3 : Inport  Port=3  OutDataTypeStr=single
  MLIB_Mac_SF : S-Function  FunctionName=MLIB_Mac_SF_FLT  SFunctionDeploymentMode=off  EnableBusSupport=off
  copyright : Subsystem
      mask Display: text(10,90,'FILE:');text(10,75,'DESRIPTION:');text(10,60,'COPYRIGHT:');text(10,45,'VERSION:');text(10,30,'DATE:')
  copyright2 : Subsystem
      mask Display: text(10,90,'MLIB_Mac_BAM_FLT.mdl');text(10,75,'Multiply-accumulte.');text(10,60,'NXP 2020');text(10,45,'1.0');text(10,30,'18-Mar-2020');
  fltOut : Outport
  wires:
  MLIB_Mac_SF/1 -> fltOut/1
  fltIn3/1 -> MLIB_Mac_SF/3
  fltIn2/1 -> MLIB_Mac_SF/2
  fltIn1/1 -> MLIB_Mac_SF/1

== system ammclib_bam/MLIB/FLT/MLIB_Mnac_FLT ==
  fltIn1 : Inport  OutDataTypeStr=single
  fltIn2 : Inport  Port=2  OutDataTypeStr=single
  fltIn3 : Inport  Port=3  OutDataTypeStr=single
  MLIB_Mnac_SF : S-Function  FunctionName=MLIB_Mnac_SF_FLT  SFunctionDeploymentMode=off  EnableBusSupport=off
  copyright : Subsystem
      mask Display: text(10,90,'FILE:');text(10,75,'DESRIPTION:');text(10,60,'COPYRIGHT:');text(10,45,'VERSION:');text(10,30,'DATE:')
  copyright2 : Subsystem
      mask Display: text(10,90,'MLIB_Mnac_BAM_FLT.mdl');text(10,75,'Multiply-negative-accumulate.');text(10,60,'NXP 2020');text(10,45,'1.0');text(10,30,'18-Mar-2020');
  fltOut : Outport
  wires:
  MLIB_Mnac_SF/1 -> fltOut/1
  fltIn3/1 -> MLIB_Mnac_SF/3
  fltIn2/1 -> MLIB_Mnac_SF/2
  fltIn1/1 -> MLIB_Mnac_SF/1

== system ammclib_bam/MLIB/FLT/MLIB_Msu_FLT ==
  fltIn1 : Inport  OutDataTypeStr=single
  fltIn2 : Inport  Port=2  OutDataTypeStr=single
  fltIn3 : Inport  Port=3  OutDataTypeStr=single
  MLIB_Msu_SF : S-Function  FunctionName=MLIB_Msu_SF_FLT  SFunctionDeploymentMode=off  EnableBusSupport=off
  copyright : Subsystem
      mask Display: text(10,90,'FILE:');text(10,75,'DESRIPTION:');text(10,60,'COPYRIGHT:');text(10,45,'VERSION:');text(10,30,'DATE:')
  copyright2 : Subsystem
      mask Display: text(10,90,'MLIB_Msu_BAM_FLT.mdl');text(10,75,'Multiply-subtract-from.');text(10,60,'NXP 2020');text(10,45,'1.0');text(10,30,'18-Mar-2020');
  fltOut : Outport
  wires:
  MLIB_Msu_SF/1 -> fltOut/1
  fltIn3/1 -> MLIB_Msu_SF/3
  fltIn2/1 -> MLIB_Msu_SF/2
  fltIn1/1 -> MLIB_Msu_SF/1

== system ammclib_bam/MLIB/FLT/MLIB_Mul_FLT ==
  fltIn1 : Inport  OutDataTypeStr=single
  fltIn2 : Inport  Port=2  OutDataTypeStr=single
  MLIB_Mul_SF : S-Function  FunctionName=MLIB_Mul_SF_FLT  SFunctionDeploymentMode=off  EnableBusSupport=off
  copyright : Subsystem
      mask Display: text(10,90,'FILE:');text(10,75,'DESRIPTION:');text(10,60,'COPYRIGHT:');text(10,45,'VERSION:');text(10,30,'DATE:')
  copyright2 : Subsystem
      mask Display: text(10,90,'MLIB_Mul_BAM_FLT.mdl');text(10,75,'Multiplication.');text(10,60,'NXP 2020');text(10,45,'1.0');text(10,30,'18-Mar-2020');
  fltOut : Outport
  wires:
  MLIB_Mul_SF/1 -> fltOut/1
  fltIn2/1 -> MLIB_Mul_SF/2
  fltIn1/1 -> MLIB_Mul_SF/1

== system ammclib_bam/MLIB/FLT/MLIB_Neg_FLT ==
  fltIn : Inport  OutDataTypeStr=single
  MLIB_Neg_SF : S-Function  FunctionName=MLIB_Neg_SF_FLT  SFunctionDeploymentMode=off  EnableBusSupport=off
  copyright : Subsystem
      mask Display: text(10,90,'FILE:');text(10,75,'DESRIPTION:');text(10,60,'COPYRIGHT:');text(10,45,'VERSION:');text(10,30,'DATE:')
  copyright2 : Subsystem
      mask Display: text(10,90,'MLIB_Neg_BAM_FLT.mdl');text(10,75,'Negation.');text(10,60,'NXP 2020');text(10,45,'1.0');text(10,30,'18-Mar-2020');
  fltOut : Outport
  wires:
  MLIB_Neg_SF/1 -> fltOut/1
  fltIn/1 -> MLIB_Neg_SF/1

== system ammclib_bam/MLIB/FLT/MLIB_Sub_FLT ==
  fltIn1 : Inport  OutDataTypeStr=single
  fltIn2 : Inport  Port=2  OutDataTypeStr=single
  MLIB_Sub_SF : S-Function  FunctionName=MLIB_Sub_SF_FLT  SFunctionDeploymentMode=off  EnableBusSupport=off
  copyright : Subsystem
      mask Display: text(10,90,'FILE:');text(10,75,'DESRIPTION:');text(10,60,'COPYRIGHT:');text(10,45,'VERSION:');text(10,30,'DATE:')
  copyright2 : Subsystem
      mask Display: text(10,90,'MLIB_Sub_BAM_FLT.mdl');text(10,75,'Subtraction.');text(10,60,'NXP 2020');text(10,45,'1.0');text(10,30,'18-Mar-2020');
  fltOut : Outport
  wires:
  MLIB_Sub_SF/1 -> fltOut/1
  fltIn2/1 -> MLIB_Sub_SF/2
  fltIn1/1 -> MLIB_Sub_SF/1

== system ammclib_bam/MLIB/FLT/MLIB_VMac_FLT ==
  fltIn1 : Inport  OutDataTypeStr=single
  fltIn2 : Inport  Port=2  OutDataTypeStr=single
  fltIn3 : Inport  Port=3  OutDataTypeStr=single
  fltIn4 : Inport  Port=4  OutDataTypeStr=single
  MLIB_VMac_SF : S-Function  FunctionName=MLIB_VMac_SF_FLT  SFunctionDeploymentMode=off  EnableBusSupport=off
  copyright : Subsystem
      mask Display: text(10,90,'FILE:');text(10,75,'DESRIPTION:');text(10,60,'COPYRIGHT:');text(10,45,'VERSION:');text(10,30,'DATE:')
  copyright2 : Subsystem
      mask Display: text(10,90,'MLIB_VMac_BAM_FLT.mdl');text(10,75,'Dot product of 2-element vectors.');text(10,60,'NXP 2020');text(10,45,'1.0');text(10,30,'18-Mar-2020');
  fltOut : Outport
  wires:
  MLIB_VMac_SF/1 -> fltOut/1
  fltIn4/1 -> MLIB_VMac_SF/4
  fltIn3/1 -> MLIB_VMac_SF/3
  fltIn2/1 -> MLIB_VMac_SF/2
  fltIn1/1 -> MLIB_VMac_SF/1

== system ammclib_bam/AMCLIB/F16/AMCLIB_BemfObsrvDQ_F16/copyright ==

== system ammclib_bam/AMCLIB/F16/AMCLIB_BemfObsrvDQ_F16/copyright2 ==

== system ammclib_bam/AMCLIB/F16/AMCLIB_CurrentLoop_F16/copyright ==

== system ammclib_bam/AMCLIB/F16/AMCLIB_CurrentLoop_F16/copyright2 ==

== system ammclib_bam/AMCLIB/F16/AMCLIB_FWSpeedLoop_F16/copyright ==

== system ammclib_bam/AMCLIB/F16/AMCLIB_FWSpeedLoop_F16/copyright2 ==

== system ammclib_bam/AMCLIB/F16/AMCLIB_FW_F16/copyright ==

== system ammclib_bam/AMCLIB/F16/AMCLIB_FW_F16/copyright2 ==

== system ammclib_bam/AMCLIB/F16/AMCLIB_SpeedLoop_F16/copyright ==

== system ammclib_bam/AMCLIB/F16/AMCLIB_SpeedLoop_F16/copyright2 ==

== system ammclib_bam/AMCLIB/F16/AMCLIB_TrackObsrv_F16/copyright ==

== system ammclib_bam/AMCLIB/F16/AMCLIB_TrackObsrv_F16/copyright2 ==

== system ammclib_bam/AMCLIB/F16/AMCLIB_Windmilling_F16/copyright ==

== system ammclib_bam/AMCLIB/F16/AMCLIB_Windmilling_F16/copyright2 ==

== system ammclib_bam/AMCLIB/F32/AMCLIB_BemfObsrvDQ_F32/copyright ==

== system ammclib_bam/AMCLIB/F32/AMCLIB_BemfObsrvDQ_F32/copyright2 ==

== system ammclib_bam/AMCLIB/F32/AMCLIB_CurrentLoop_F32/copyright ==

== system ammclib_bam/AMCLIB/F32/AMCLIB_CurrentLoop_F32/copyright2 ==

== system ammclib_bam/AMCLIB/F32/AMCLIB_FWSpeedLoop_F32/copyright ==

== system ammclib_bam/AMCLIB/F32/AMCLIB_FWSpeedLoop_F32/copyright2 ==

== system ammclib_bam/AMCLIB/F32/AMCLIB_FW_F32/copyright ==

== system ammclib_bam/AMCLIB/F32/AMCLIB_FW_F32/copyright2 ==

== system ammclib_bam/AMCLIB/F32/AMCLIB_SpeedLoop_F32/copyright ==

== system ammclib_bam/AMCLIB/F32/AMCLIB_SpeedLoop_F32/copyright2 ==

== system ammclib_bam/AMCLIB/F32/AMCLIB_TrackObsrv_F32/copyright ==

== system ammclib_bam/AMCLIB/F32/AMCLIB_TrackObsrv_F32/copyright2 ==

== system ammclib_bam/AMCLIB/F32/AMCLIB_Windmilling_F32/copyright ==

== system ammclib_bam/AMCLIB/F32/AMCLIB_Windmilling_F32/copyright2 ==

== system ammclib_bam/AMCLIB/FLT/AMCLIB_BemfObsrvDQ_FLT/copyright ==

== system ammclib_bam/AMCLIB/FLT/AMCLIB_BemfObsrvDQ_FLT/copyright2 ==

== system ammclib_bam/AMCLIB/FLT/AMCLIB_CurrentLoop_FLT/copyright ==

== system ammclib_bam/AMCLIB/FLT/AMCLIB_CurrentLoop_FLT/copyright2 ==

== system ammclib_bam/AMCLIB/FLT/AMCLIB_FWSpeedLoop_FLT/copyright ==

== system ammclib_bam/AMCLIB/FLT/AMCLIB_FWSpeedLoop_FLT/copyright2 ==

== system ammclib_bam/AMCLIB/FLT/AMCLIB_FW_FLT/copyright ==

== system ammclib_bam/AMCLIB/FLT/AMCLIB_FW_FLT/copyright2 ==

== system ammclib_bam/AMCLIB/FLT/AMCLIB_SpeedLoop_FLT/copyright ==

== system ammclib_bam/AMCLIB/FLT/AMCLIB_SpeedLoop_FLT/copyright2 ==

== system ammclib_bam/AMCLIB/FLT/AMCLIB_TrackObsrv_FLT/copyright ==

== system ammclib_bam/AMCLIB/FLT/AMCLIB_TrackObsrv_FLT/copyright2 ==

== system ammclib_bam/AMCLIB/FLT/AMCLIB_Windmilling_FLT/copyright ==

== system ammclib_bam/AMCLIB/FLT/AMCLIB_Windmilling_FLT/copyright2 ==

== system ammclib_bam/GDFLIB/F16/GDFLIB_FilterFIR_F16/copyright ==

== system ammclib_bam/GDFLIB/F16/GDFLIB_FilterFIR_F16/copyright2 ==

== system ammclib_bam/GDFLIB/F16/GDFLIB_FilterIIR1_F16/copyright ==

== system ammclib_bam/GDFLIB/F16/GDFLIB_FilterIIR1_F16/copyright2 ==

== system ammclib_bam/GDFLIB/F16/GDFLIB_FilterIIR2_F16/copyright ==

== system ammclib_bam/GDFLIB/F16/GDFLIB_FilterIIR2_F16/copyright2 ==

== system ammclib_bam/GDFLIB/F16/GDFLIB_FilterMA_F16/copyright ==

== system ammclib_bam/GDFLIB/F16/GDFLIB_FilterMA_F16/copyright2 ==

== system ammclib_bam/GDFLIB/F32/GDFLIB_FilterFIR_F32/copyright ==

== system ammclib_bam/GDFLIB/F32/GDFLIB_FilterFIR_F32/copyright2 ==

== system ammclib_bam/GDFLIB/F32/GDFLIB_FilterIIR1_F32/copyright ==

== system ammclib_bam/GDFLIB/F32/GDFLIB_FilterIIR1_F32/copyright2 ==

== system ammclib_bam/GDFLIB/F32/GDFLIB_FilterIIR2_F32/copyright ==

== system ammclib_bam/GDFLIB/F32/GDFLIB_FilterIIR2_F32/copyright2 ==

== system ammclib_bam/GDFLIB/F32/GDFLIB_FilterMA_F32/copyright ==

== system ammclib_bam/GDFLIB/F32/GDFLIB_FilterMA_F32/copyright2 ==

== system ammclib_bam/GDFLIB/FLT/GDFLIB_FilterFIR_FLT/copyright ==

== system ammclib_bam/GDFLIB/FLT/GDFLIB_FilterFIR_FLT/copyright2 ==

== system ammclib_bam/GDFLIB/FLT/GDFLIB_FilterIIR1_FLT/copyright ==

== system ammclib_bam/GDFLIB/FLT/GDFLIB_FilterIIR1_FLT/copyright2 ==

== system ammclib_bam/GDFLIB/FLT/GDFLIB_FilterIIR2_FLT/copyright ==

== system ammclib_bam/GDFLIB/FLT/GDFLIB_FilterIIR2_FLT/copyright2 ==

== system ammclib_bam/GDFLIB/FLT/GDFLIB_FilterMA_FLT/copyright ==

== system ammclib_bam/GDFLIB/FLT/GDFLIB_FilterMA_FLT/copyright2 ==

== system ammclib_bam/GFLIB/F16/GFLIB_Acos_F16/copyright ==

== system ammclib_bam/GFLIB/F16/GFLIB_Acos_F16/copyright2 ==

== system ammclib_bam/GFLIB/F16/GFLIB_Asin_F16/copyright ==

== system ammclib_bam/GFLIB/F16/GFLIB_Asin_F16/copyright2 ==

== system ammclib_bam/GFLIB/F16/GFLIB_AtanYXShifted_F16/copyright ==

== system ammclib_bam/GFLIB/F16/GFLIB_AtanYXShifted_F16/copyright2 ==

== system ammclib_bam/GFLIB/F16/GFLIB_AtanYX_F16/copyright ==

== system ammclib_bam/GFLIB/F16/GFLIB_AtanYX_F16/copyright2 ==

== system ammclib_bam/GFLIB/F16/GFLIB_Atan_F16/copyright ==

== system ammclib_bam/GFLIB/F16/GFLIB_Atan_F16/copyright2 ==

== system ammclib_bam/GFLIB/F16/GFLIB_ControllerPIDpAW_F16/copyright ==

== system ammclib_bam/GFLIB/F16/GFLIB_ControllerPIDpAW_F16/copyright2 ==

== system ammclib_bam/GFLIB/F16/GFLIB_ControllerPIpAW_F16/copyright ==

== system ammclib_bam/GFLIB/F16/GFLIB_ControllerPIpAW_F16/copyright2 ==

== system ammclib_bam/GFLIB/F16/GFLIB_ControllerPIp_F16/copyright ==

== system ammclib_bam/GFLIB/F16/GFLIB_ControllerPIp_F16/copyright2 ==

== system ammclib_bam/GFLIB/F16/GFLIB_ControllerPIrAW_F16/copyright ==

== system ammclib_bam/GFLIB/F16/GFLIB_ControllerPIrAW_F16/copyright2 ==

== system ammclib_bam/GFLIB/F16/GFLIB_ControllerPIr_F16/copyright ==

== system ammclib_bam/GFLIB/F16/GFLIB_ControllerPIr_F16/copyright2 ==

== system ammclib_bam/GFLIB/F16/GFLIB_Cos_F16/copyright ==

== system ammclib_bam/GFLIB/F16/GFLIB_Cos_F16/copyright2 ==

== system ammclib_bam/GFLIB/F16/GFLIB_Hyst_F16/copyright ==

== system ammclib_bam/GFLIB/F16/GFLIB_Hyst_F16/copyright2 ==

== system ammclib_bam/GFLIB/F16/GFLIB_IntegratorTR_F16/copyright ==

== system ammclib_bam/GFLIB/F16/GFLIB_IntegratorTR_F16/copyright2 ==

== system ammclib_bam/GFLIB/F16/GFLIB_Limit_F16/copyright ==

== system ammclib_bam/GFLIB/F16/GFLIB_Limit_F16/copyright2 ==

== system ammclib_bam/GFLIB/F16/GFLIB_LowerLimit_F16/copyright ==

== system ammclib_bam/GFLIB/F16/GFLIB_LowerLimit_F16/copyright2 ==

== system ammclib_bam/GFLIB/F16/GFLIB_Lut1D_F16/copyright ==

== system ammclib_bam/GFLIB/F16/GFLIB_Lut1D_F16/copyright2 ==

== system ammclib_bam/GFLIB/F16/GFLIB_Lut2D_F16/copyright ==

== system ammclib_bam/GFLIB/F16/GFLIB_Lut2D_F16/copyright2 ==

== system ammclib_bam/GFLIB/F16/GFLIB_Ramp_F16/copyright ==

== system ammclib_bam/GFLIB/F16/GFLIB_Ramp_F16/copyright2 ==

== system ammclib_bam/GFLIB/F16/GFLIB_Sign_F16/copyright ==

== system ammclib_bam/GFLIB/F16/GFLIB_Sign_F16/copyright2 ==

== system ammclib_bam/GFLIB/F16/GFLIB_SinCos_F16/copyright ==

== system ammclib_bam/GFLIB/F16/GFLIB_SinCos_F16/copyright2 ==

== system ammclib_bam/GFLIB/F16/GFLIB_Sin_F16/copyright ==

== system ammclib_bam/GFLIB/F16/GFLIB_Sin_F16/copyright2 ==

== system ammclib_bam/GFLIB/F16/GFLIB_Sqrt_F16/copyright ==

== system ammclib_bam/GFLIB/F16/GFLIB_Sqrt_F16/copyright2 ==

== system ammclib_bam/GFLIB/F16/GFLIB_Tan_F16/copyright ==

== system ammclib_bam/GFLIB/F16/GFLIB_Tan_F16/copyright2 ==

== system ammclib_bam/GFLIB/F16/GFLIB_UpperLimit_F16/copyright ==

== system ammclib_bam/GFLIB/F16/GFLIB_UpperLimit_F16/copyright2 ==

== system ammclib_bam/GFLIB/F16/GFLIB_VMin_F16/copyright ==

== system ammclib_bam/GFLIB/F16/GFLIB_VMin_F16/copyright2 ==

== system ammclib_bam/GFLIB/F16/GFLIB_VectorLimit_F16/copyright ==

== system ammclib_bam/GFLIB/F16/GFLIB_VectorLimit_F16/copyright2 ==

== system ammclib_bam/GFLIB/F32/GFLIB_Acos_F32/copyright ==

== system ammclib_bam/GFLIB/F32/GFLIB_Acos_F32/copyright2 ==

== system ammclib_bam/GFLIB/F32/GFLIB_Asin_F32/copyright ==

== system ammclib_bam/GFLIB/F32/GFLIB_Asin_F32/copyright2 ==

== system ammclib_bam/GFLIB/F32/GFLIB_AtanYXShifted_F32/copyright ==

== system ammclib_bam/GFLIB/F32/GFLIB_AtanYXShifted_F32/copyright2 ==

== system ammclib_bam/GFLIB/F32/GFLIB_AtanYX_F32/copyright ==

== system ammclib_bam/GFLIB/F32/GFLIB_AtanYX_F32/copyright2 ==

== system ammclib_bam/GFLIB/F32/GFLIB_Atan_F32/copyright ==
